simulink model "VOO"  (R2020a)
settings: Solver=FixedStepAuto  StartTime=0.0  StopTime=10.0  FixedStep=1e-3  RelTol=1e-3  EnableMultiTasking=on
undefined symbols (not defined in the file): D10, D12, D2, D5, D7, D9, PTA2, PTB9, PTC3, PTC4, PTD0, PTD3
libraries: frdmk64flib x8
settings Model: ExtModeTrigDuration=5  Creator=karir  LastModifiedBy=karir
settings OptimizationCC: EnhancedBackFolding=on  PassReuseOutputArgsAs=Individual arguments  ZeroExternalMemoryAtStartup=off  ZeroInternalMemoryAtStartup=off  MaxStackSize=64  OptimizeBlockOrder=speed  DifferentSizesBufferReuse=on  OptimizationCustomize=off  EfficientTunableParamExpr=on
settings DebuggingCC: ParameterTunabilityLossMsg=error
settings HardwareCC: ProdBitPerPointer=32  ProdBitPerSizeT=32  ProdBitPerPtrDiffT=32  ProdLargestAtomicInteger=Long  ProdLargestAtomicFloat=Double  ProdWordSize=32  ProdHWDeviceType=ARM Compatible->ARM Cortex
settings SFSimCC: MATLABDynamicMemAlloc=off
settings RTWCC: SystemTargetFile=ert.tlc  HardwareBoard=NXP FRDM-K64F  TemplateMakefile=ert_default_tmf  Toolchain=GNU Tools for ARM Embedded Processors
settings CodeAppCC: ForceParamTrailComments=on  IgnoreCustomStorageClasses=off  OperatorAnnotations=on  SimulinkDataObjDesc=on  SFDataObjDesc=on  InsertBlockDesc=on

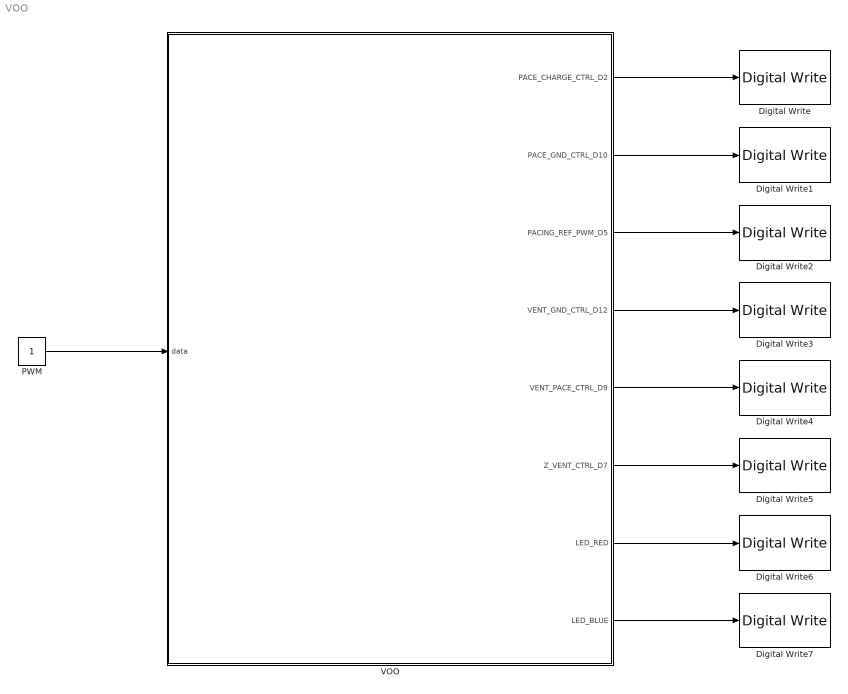
== system VOO ==
  Digital Write : frdmk64flib/Digital Write  Whichpin=PTB9 (D2)
  Digital Write1 : frdmk64flib/Digital Write  Whichpin=PTD0 (D10)
  Digital Write2 : frdmk64flib/Digital Write  Whichpin=PTA2 (D5)
  Digital Write3 : frdmk64flib/Digital Write  Whichpin=PTD3 (D12)
  Digital Write4 : frdmk64flib/Digital Write  Whichpin=PTC4 (D9)
  Digital Write5 : frdmk64flib/Digital Write  Whichpin=PTC3 (D7)
  Digital Write6 : frdmk64flib/Digital Write  Whichpin=RED_LED
  Digital Write7 : frdmk64flib/Digital Write  Whichpin=BLUE_LED
  PWM : Constant
  VOO : Stateflow chart  TreatAsAtomicUnit=on
  wires:
  PWM/1 -> VOO/1(data)
  VOO/1(PACE_CHARGE_CTRL_D2) -> Digital Write/1
  VOO/2(PACE_GND_CTRL_D10) -> Digital Write1/1
  VOO/3(PACING_REF_PWM_D5) -> Digital Write2/1
  VOO/4(VENT_GND_CTRL_D12) -> Digital Write3/1
  VOO/5(VENT_PACE_CTRL_D9) -> Digital Write4/1
  VOO/6(Z_VENT_CTRL_D7) -> Digital Write5/1
  VOO/7(LED_RED) -> Digital Write6/1
  VOO/8(LED_BLUE) -> Digital Write7/1

== stateflow chart VOO/VOO ==
  state Charging
    entry:
    PACING_REF_PWM_D5 = data;
    PACE_CHARGE_CTRL_D2 = 1;
    VENT_PACE_CTRL_D9 = 0;
    VENT_GND_CTRL_D12 = 1;
    PACE_GND_CTRL_D10 = 0;
    Z_VENT_CTRL_D7 = 0;
    LED_RED = 0;
    LED_BLUE = 1;
  state Pacing
    entry:
    PACING_REF_PWM_D5 = data;
    PACE_CHARGE_CTRL_D2 = 0;
    VENT_PACE_CTRL_D9 = 1;
    VENT_GND_CTRL_D12 = 0;
    PACE_GND_CTRL_D10 = 1;
    Z_VENT_CTRL_D7 = 0;
    LED_RED = 1;
    LED_BLUE = 0;
  (default) -> Charging
  Charging -> Pacing : [after(980,msec)]
  Pacing -> Charging : [after(20,msec)]
  data: data input; PACE_CHARGE_CTRL_D2 output; PACE_GND_CTRL_D10 output; PACING_REF_PWM_D5 output; VENT_GND_CTRL_D12 output; VENT_PACE_CTRL_D9 output; Z_VENT_CTRL_D7 output; LED_RED output; LED_BLUE output
